simulink model "mdlepimol"  (Simulink 7.8)
settings: Solver=ode45  StartTime=0.0  StopTime=10  RelTol=1e-3
settings Model: Creator=klempond  LastModifiedBy=polacekm
settings GRTTargetCC: CombineOutputUpdateFcns=on

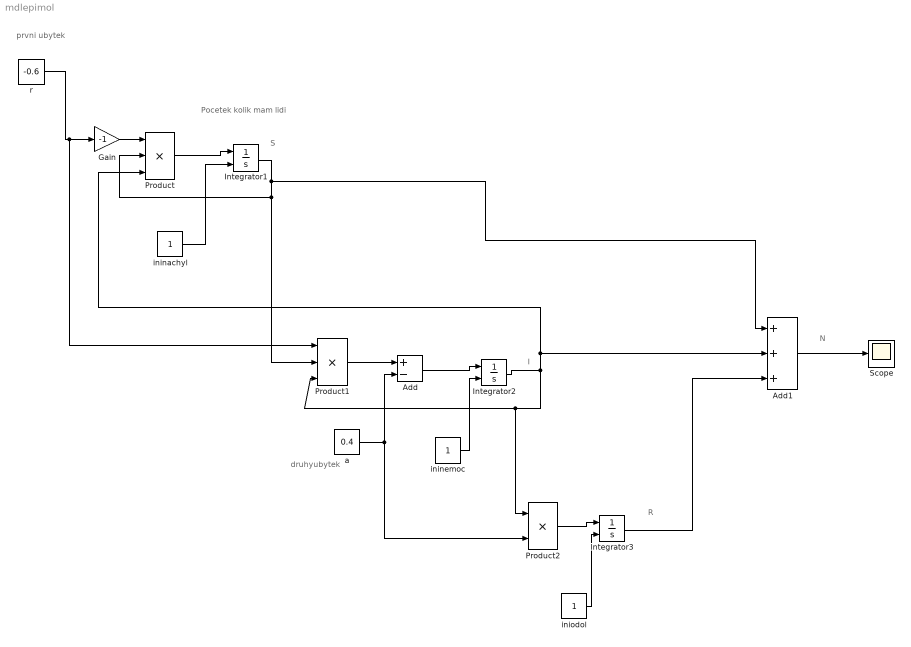
== system mdlepimol ==
  note: S
  note: I
  note: R
  note: N
  note: Pocetek kolik mam lidi
  note: prvni ubytek
  note: druhyubytek
  Add : Sum  Inputs=+-
  Add1 : Sum  Inputs=+++
  Gain : Gain  Gain=-1
  Integrator1 : Integrator  InitialConditionSource=external  InitialCondition=100
  Integrator2 : Integrator  InitialConditionSource=external  InitialCondition=1
  Integrator3 : Integrator  InitialConditionSource=external  InitialCondition=1
  Product : Product  Inputs=3  RndMeth=Zero
  Product1 : Product  Inputs=3  RndMeth=Zero
  Product2 : Product  RndMeth=Zero
  Scope : Scope
      settings: SaveName=sc
  a : Constant  Value=0.4
  ininachyl : Constant
  ininemoc : Constant
  iniodol : Constant
  r : Constant  Value=-0.6
  wires:
  Product/1 -> Integrator1/1
  Gain/1 -> Product/1
  r/1 -> Gain/1, Product1/1
  Integrator1/1 -> Product/2, Product1/2, Add1/1
  Integrator2/1 -> Product1/3, Product2/1, Product/3, Add1/2
  Product1/1 -> Add/1
  a/1 -> Add/2, Product2/2
  Add/1 -> Integrator2/1
  Product2/1 -> Integrator3/1
  Integrator3/1 -> Add1/3
  Add1/1 -> Scope/1
  ininachyl/1 -> Integrator1/2
  ininemoc/1 -> Integrator2/2
  iniodol/1 -> Integrator3/2
